simulink model "rtwdemo_dynamicio"  (Simulink 7.6)
settings: Solver=FixedStepDiscrete  StartTime=0.0  StopTime=1  FixedStep=1  RelTol=1e-3
PostLoadFcn:
  | clear;K=Simulink.Parameter;K.Value=2;K.RTWInfo.StorageClass='SimulinkGlobal';
libraries: rtwdemowidgets x2
Description:
  | Sharing Data Among Simulink(R), Stateflow(R), and Embedded MATLAB(TM)
settings Model: Creator=The MathWorks Inc.  ExtModeAutoUpdateStatusClock=off
settings MATStruct: SampleTime=1  Offset=0  Priority=[20.0]
settings DataIOCC: LimitDataPoints=off  SaveOutput=off  SaveTime=off  SignalLoggingName=logsOut
settings OptimizationCC: InlineParams=on  InlineInvariantSignals=on  StateBitsets=on  DataBitsets=on  UseTempVars=on  EfficientFloat2IntCast=on  EfficientMapNaN2IntZero=off
settings DebuggingCC: CheckExecutionContextPreStartOutputMsg=on  CheckExecutionContextRuntimeOutputMsg=on  SolverPrmCheckMsg=none  StrictBusMsg=ErrorOnBusTreatedAsVector
settings HardwareCC: ProdIntDivRoundTo=Zero  ProdEndianess=LittleEndian  ProdHWDeviceType=Generic->32-bit Embedded Processor  TargetHWDeviceType=Generic->32-bit Embedded Processor
settings ModelReferenceCC: UpdateModelReferenceTargets=IfOutOfDate
settings SFSimCC: SimParseCustomCode=off
settings RTWCC: Description=RTW Embedded Coder (no auto configuration)  GenerateReport=on  RTWVerbose=off  ProcessScript=grt_make_rtw_hook  LaunchReport=on
settings CodeAppCC: ForceParamTrailComments=on
settings GRTTargetCC: TargetFcnLib=ansi_tfl_tmw.mat

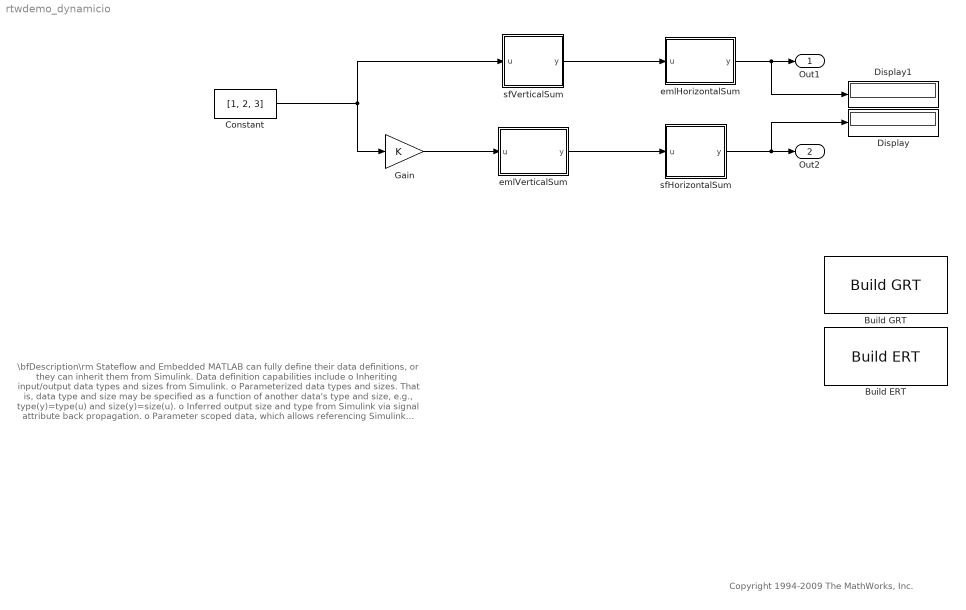
== system rtwdemo_dynamicio ==
  note: \bfDescription\rm
      | Stateflow and Embedded MATLAB can fully define their data definitions, or they can
      | inherit them from Simulink.  Data definition capabilities include
      |
      | o Inheriting input/output data types and sizes from Simulink.
      | o Parameterized data types and sizes.  That is, data type and size may be specified
      |    as a function of another data's type and size, e.g., type(y)=type(u) and size(y)=size(u).
      | o Inferred output size and type from Simulink via signal attribute back propagation.
      | o Parameter scoped data, which allows referencing Simulink parameters in Stateflow and
      |    Embedded MATLAB.
      |
      | \bfInstructions\rm
      | o Compile the model (Edit > Update Diagram) and note the displayed signal types and sizes.
      | o Change the data type and/or size of the Constant block and recompile the model.  Note
      |    that the attributes of the signals automatically adapt to the Constant block specification.
      | o Generate and inspect code using the blue buttons to the right.  Note that K is shared
      |    by the Gain and sfVerticalSum block.
      |
      | \bfNotes\rm
      | o The data type and size of all Stateflow and Embedded MATLAB data is inherited from Simulink.
      | o The Gain block and the Stateflow chart sfVerticalSum share the Simulink parameter K, which is
      |    defined in the MATLAB workspace as a Simulink.Parameter with SimulinkGlobal storage
      |    class (i.e., rtP.K in the generated code).
  note: Copyright 1994-2009 The MathWorks, Inc.
  Build ERT : rtwdemowidgets/Build ERT  SystemSampleTime=-1  attrib_overrides={}
  Build GRT : rtwdemowidgets/Build GRT  SystemSampleTime=-1  attrib_overrides={}
  Constant : Constant  Value=[1, 2, 3]  VectorParams1D=off  OutDataTypeStr=single
  Display : Display
  Display1 : Display
  Gain : Gain  Gain=K  OutDataTypeStr=Inherit: Same as input  ParamDataTypeStr=Inherit: Same as input
  emlHorizontalSum : Stateflow chart  TreatAsAtomicUnit=on
  emlVerticalSum : Stateflow chart  TreatAsAtomicUnit=on
  sfHorizontalSum : Stateflow chart  TreatAsAtomicUnit=on
  sfVerticalSum : Stateflow chart  TreatAsAtomicUnit=on
  Out1 : Outport
  Out2 : Outport  Port=2
  wires:
  emlVerticalSum/1(y) -> sfHorizontalSum/1(u)
  sfHorizontalSum/1(y) -> Out2/1, Display/1
  sfVerticalSum/1(y) -> emlHorizontalSum/1(u)
  emlHorizontalSum/1(y) -> Out1/1, Display1/1
  Gain/1 -> emlVerticalSum/1(u)
  Constant/1 -> sfVerticalSum/1(u), Gain/1

== matlab function emlHorizontalSum ==
  data: u input double; y output type(u)
function y = fcn(u)
y = sum(u,2);

== matlab function emlVerticalSum ==
  data: u input double; y output type(u)
function y = fcn(u)
y = sum(u,1);

== matlab function sfHorizontalSum ==
  data: u1 function_input type(u) size=size(u); y1 function_output type(u) size=[size(u,1) 1]; u input double; y output type(u) size=[size(u,1),1]
function y1 = f(u1)
y1 = sum(u1,2);

== matlab function sfVerticalSum ==
  data: u1 function_input type(u) size=size(u); y1 function_output type(u) size=[1 size(u,2)]; u input double; y output type(u) size=[1,size(u,2)]; K parameter type(u)
function y1 = f(u1)
y1 = sum(u1,1);
